simulink model "SimToStewartPlatform"  (R2020a)
settings: Solver=VariableStepAuto  StartTime=0.0  StopTime=inf  RelTol=1e-3
undefined symbols (not defined in the file or in its folder): Standard_Devices, UDP_Protocol
libraries: eeGeneralControl x3, instrumentlib x3, sldrtlib x1, simulink x1, ptplib x1
settings Model: xpc_rtwmakecfg_data=_xpcetherlib__xpcether8255xlib__xpcetherGbElib__xpciplib__xpcnblib_  Creator=meta_  LastModifiedBy=filip

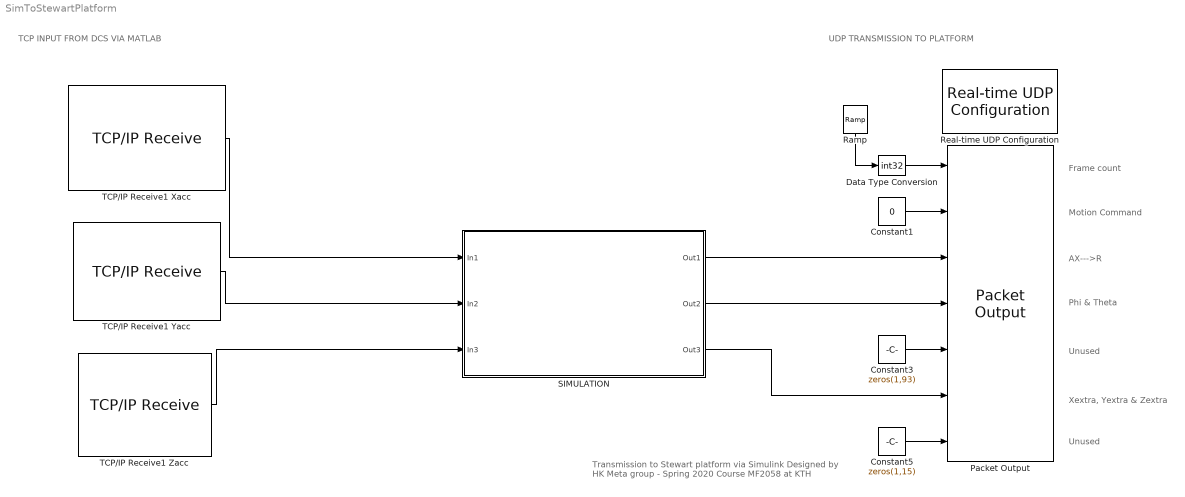
== system SimToStewartPlatform ==
  note: Transmission to Stewart platform via Simulink
      | Designed by HK Meta group - Spring 2020
      | Course MF2058 at KTH
  note: TCP INPUT FROM DCS VIA MATLAB
  note: UDP TRANSMISSION TO PLATFORM
  note: Unused
  note: Frame count
  note: Unused
  note: Phi & Theta
  note: Motion Command
  note: AX--->R
  note: Xextra, Yextra & Zextra
  Constant1 : Constant  Value=0
  Constant3 : Constant  Value=zeros(1,93)
  Constant5 : Constant  Value=zeros(1,15)
  Data Type Conversion : DataTypeConversion  OutDataTypeStr=int32
  Packet Output : sldrtlib/Packet Output  SampleTime=0.1  MaxMissedTicks=inf  ShowMissedTicks=off  YieldWhenWaiting=on  DrvName=Standard_Devices/UDP_Protocol  DrvAddress=16384  DrvOptions=[0 16385 49 57 50 46 49 54 56 46 57 48 46 50 52 48 0 0 0 0 0 0 0 0 0 0 0 0 0 0 0 0 0 0 0 0 0 0 0 0 0 0 0 0 0 0 0 0 0 0 0 0 0 0 0 0 0 0 0 0 0 0 0 0 0 0 0 0 0 0 0 0 0 0 0 0 0 0 0 0 0 0 0 0 0 0 0 0 0 0 0 0 0 0 0 0 0 0 0 0 0 0 0 0 0 0 0 0 0 0 0 0 0 0 0 0 0 0 0 0 0 0 0 0 0 0 0 0 0 0 0 0 0 0 0 0 0 0 0 0 0 0 0 0 0 0 0 0 0 0 0 0 0 0 0 0 0 0 0 0 0 0 0 0 0 0 0 0 0 0 0 0 0 0 0 0 0 0 0 0 0 0 0 0 0 0 0 0 0 0 0 0 0 0 0 0 0 0 0 0 0 0 0 0 0 0 0 0 0 0 0 0 0 0 0 0 0 0 0 0 0 0 0 0 0 0 0 0 0 0 0 0 0 0 0 0 0 0 0 0 0 0 0 0 0 0 0 0 0 0 0 0 0 0 0 0]  PacketSize=508  DataTypes={'1*int32','1*int32','12*single','2*single','93*single','3*single','15*single'}  ShowReady=off  ShowError=off  PacketID=1  ByteOrder=1  InitialValue=[]  FinalValue=[]
      settings: AttributesFormatString=UDP Protocol [16384]
  Ramp : simulink/Sources/Ramp  slope=10  start=0  InitialOutput=0
  "Real-time UDP Configuration " : ptplib/PTP UDP/Real-time UDP  Configuration   ID=1  IpAddress=192.168.90.241  SubnetMask=255.255.255.0  Gateway=0.0.0.0  EthDrv=Intel Gigabit  PciBus=0  PciSlot=31  PciFunction=6  udpID=0  MulticastList=[]  Multicast={}
      settings: SourceProductBaseCode=XP
  SIMULATION : Subsystem
  TCP/IP Receive1 Xacc : instrumentlib/TCP//IP Receive  Host=127.0.0.1  Port=31091  DataSize="[1  1]"  EnableBlockingMode=on  Timeout=10  SampleTime=0.01  DataType=ASCII  ByteOrder=BigEndian  ASCIIFormatting=%f  Terminator=LF
  TCP/IP Receive1 Yacc : instrumentlib/TCP//IP Receive  Host=127.0.0.1  Port=31092  DataSize="[1  1]"  EnableBlockingMode=on  Timeout=10  SampleTime=0.01  DataType=ASCII  ByteOrder=BigEndian  ASCIIFormatting=%f  Terminator=LF
  TCP/IP Receive1 Zacc : instrumentlib/TCP//IP Receive  Host=127.0.0.1  Port=31093  DataSize="[1  1]"  EnableBlockingMode=on  Timeout=10  SampleTime=0.01  DataType=ASCII  ByteOrder=BigEndian  ASCIIFormatting=%f  Terminator=LF
  wires:
  Data Type Conversion/1 -> Packet Output/1
  Constant5/1 -> Packet Output/7
  Constant3/1 -> Packet Output/5
  Ramp/1 -> Data Type Conversion/1
  Constant1/1 -> Packet Output/2
  TCP/IP Receive1 Xacc/1 -> SIMULATION/1(In1)
  TCP/IP Receive1 Yacc/1 -> SIMULATION/2(In2)
  TCP/IP Receive1 Zacc/1 -> SIMULATION/3(In3)
  SIMULATION/1(Out1) -> Packet Output/3
  SIMULATION/2(Out2) -> Packet Output/4
  SIMULATION/3(Out3) -> Packet Output/6

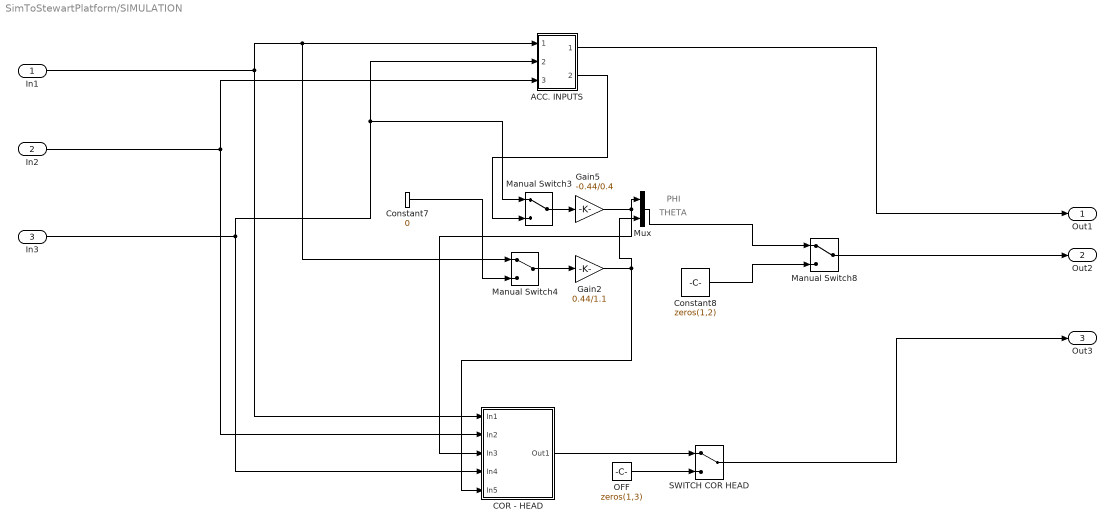
== system SimToStewartPlatform/SIMULATION ==
  note: THETA
  note: PHI
  In1 : Inport
  In2 : Inport  Port=2
  In3 : Inport  Port=3
  "ACC. INPUTS " : Subsystem
  COR - HEAD : Subsystem
  Constant7 : Constant  Value=0
  Constant8 : Constant  Value=zeros(1,2)
  Gain2 : Gain  Gain=0.44/1.1
  Gain5 : Gain  Gain=-0.44/0.4
  Manual Switch3 : ManualSwitch
  Manual Switch4 : ManualSwitch
  Manual Switch8 : ManualSwitch
  Mux : Mux  Inputs=2
  OFF : Constant  Value=zeros(1,3)
  SWITCH COR HEAD : ManualSwitch
  Out1 : Outport
  Out2 : Outport  Port=2
  Out3 : Outport  Port=3
  wires:
  COR - HEAD/1(Out1) -> SWITCH COR HEAD/1
  In1/1 -> COR - HEAD/1(In1), "ACC. INPUTS "/1(In1), Manual Switch4/1
  In3/1 -> COR - HEAD/4(In4), "ACC. INPUTS "/2(In2), Manual Switch3/1
  Gain5/1 -> COR - HEAD/3(In3), Mux/1
  Gain2/1 -> COR - HEAD/5(In5), Mux/2
  "ACC. INPUTS "/1(Out1) -> Out1/1
  Manual Switch3/1 -> Gain5/1
  Constant7/1 -> Manual Switch4/2
  Mux/1 -> Manual Switch8/1
  Constant8/1 -> Manual Switch8/2
  Manual Switch4/1 -> Gain2/1
  In2/1 -> "ACC. INPUTS "/3(In3), COR - HEAD/2(In2)
  SWITCH COR HEAD/1 -> Out3/1
  OFF/1 -> SWITCH COR HEAD/2
  "ACC. INPUTS "/2(Out2) -> Manual Switch3/2
  Manual Switch8/1 -> Out2/1

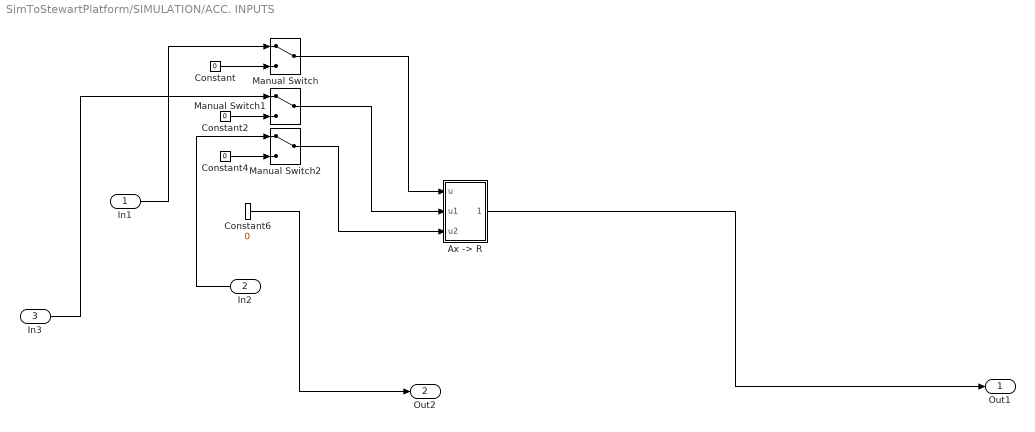
== system SimToStewartPlatform/SIMULATION/ACC. INPUTS  ==
  In1 : Inport
  In2 : Inport  Port=2
  In3 : Inport  Port=3
  "Ax -> R" : Subsystem
  Constant{,2,4,6} (4 alike) : Constant  Value=0
  Manual Switch : ManualSwitch
  Manual Switch1 : ManualSwitch
  Manual Switch2 : ManualSwitch
  Out1 : Outport
  Out2 : Outport  Port=2
  wires:
  Manual Switch2/1 -> "Ax -> R"/3(u2)
  "Ax -> R"/1(Out1) -> Out1/1
  Constant4/1 -> Manual Switch2/2
  Manual Switch/1 -> "Ax -> R"/1(u)
  Constant2/1 -> Manual Switch1/2
  In3/1 -> Manual Switch1/1
  Manual Switch1/1 -> "Ax -> R"/2(u1)
  Constant/1 -> Manual Switch/2
  In1/1 -> Manual Switch/1
  Constant6/1 -> Out2/1
  In2/1 -> Manual Switch2/1

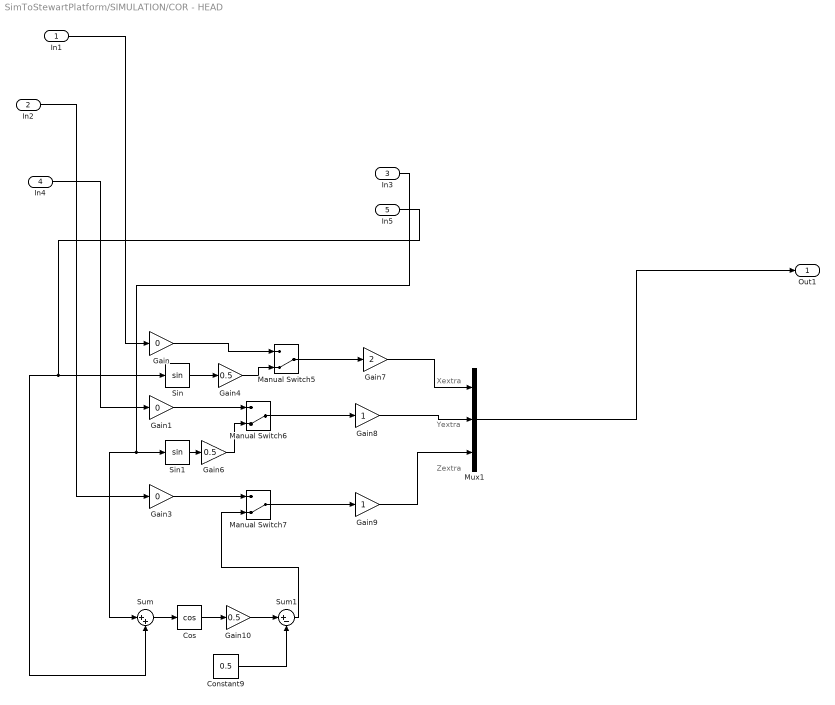
== system SimToStewartPlatform/SIMULATION/COR - HEAD ==
  note: Xextra
  note: Yextra
  note: Zextra
  In1 : Inport
  In2 : Inport  Port=2
  In3 : Inport  Port=3
  In4 : Inport  Port=4
  In5 : Inport  Port=5
  Constant9 : Constant  Value=0.5
  Cos : Trigonometry  Operator=cos
  Gain : Gain  Gain=0
  Gain1 : Gain  Gain=0
  Gain10 : Gain  Gain=0.5
  Gain3 : Gain  Gain=0
  Gain4 : Gain  Gain=0.5
  Gain6 : Gain  Gain=0.5
  Gain7 : Gain  Gain=2
  Gain8 : Gain
  Gain9 : Gain
  Manual Switch5 : ManualSwitch  CurrentSetting=0
  Manual Switch6 : ManualSwitch  CurrentSetting=0
  Manual Switch7 : ManualSwitch  CurrentSetting=0
  Mux1 : Mux  Inputs=3
  Sin : Trigonometry
  Sin1 : Trigonometry
  Sum : Sum  Inputs=|++
  Sum1 : Sum  Inputs=|+-
  Out1 : Outport
  wires:
  In3/1 -> Sum/1, Sin1/1
  Gain1/1 -> Manual Switch6/1
  In5/1 -> Sum/2, Sin/1
  Sin/1 -> Gain4/1
  Gain6/1 -> Manual Switch6/2
  Gain7/1 -> Mux1/1
  Sum/1 -> Cos/1
  Mux1/1 -> Out1/1
  Sin1/1 -> Gain6/1
  Gain/1 -> Manual Switch5/1
  Gain3/1 -> Manual Switch7/1
  Constant9/1 -> Sum1/2
  Sum1/1 -> Manual Switch7/2
  Gain9/1 -> Mux1/3
  Manual Switch5/1 -> Gain7/1
  Manual Switch7/1 -> Gain9/1
  Gain8/1 -> Mux1/2
  Cos/1 -> Gain10/1
  Gain4/1 -> Manual Switch5/2
  Manual Switch6/1 -> Gain8/1
  Gain10/1 -> Sum1/1
  In4/1 -> Gain1/1
  In2/1 -> Gain3/1
  In1/1 -> Gain/1

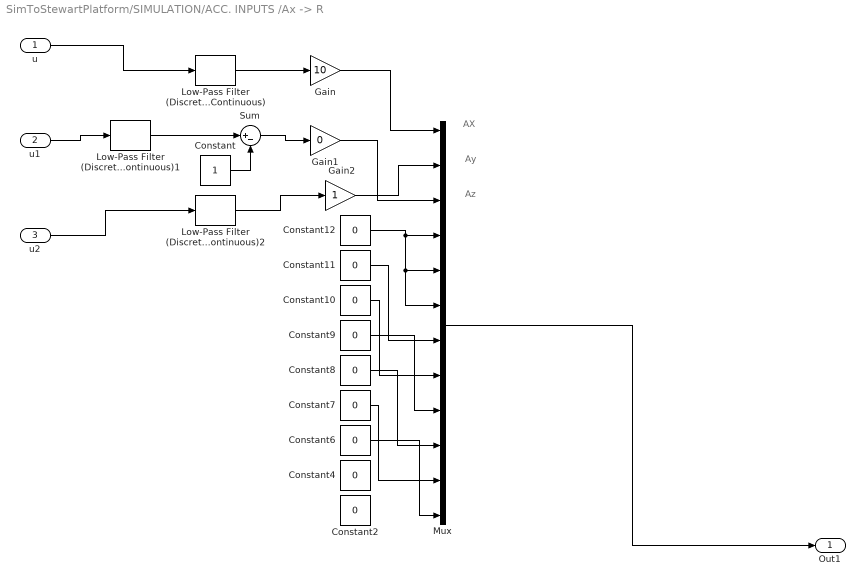
== system SimToStewartPlatform/SIMULATION/ACC. INPUTS /Ax -> R ==
  note: Az
  note: Ay
  note: AX
  u : Inport
  u1 : Inport  Port=2
  u2 : Inport  Port=3
  Constant : Constant
  Constant{2,4,6..12} (9 alike) : Constant  Value=0
  Gain : Gain  Gain=10
  Gain1 : Gain  Gain=0
  Gain2 : Gain
  Low-Pass Filter (Discrete or Continuous) : eeGeneralControl/Low-Pass Filter (Discrete or Continuous)  K=1  T=1  B=inf  A=-inf  init_option=Inherited from block input  x0=0  Ts=-1
  Low-Pass Filter (Discrete or Continuous)1 : eeGeneralControl/Low-Pass Filter (Discrete or Continuous)  K=1  T=1  B=inf  A=-inf  init_option=Inherited from block input  x0=0  Ts=-1
  Low-Pass Filter (Discrete or Continuous)2 : eeGeneralControl/Low-Pass Filter (Discrete or Continuous)  K=1  T=1  B=inf  A=-inf  init_option=Inherited from block input  x0=0  Ts=-1
  Mux : Mux  Inputs=12
  Sum : Sum  Inputs=|+-
  Out1 : Outport
  wires:
  Constant9/1 -> Mux/9
  u/1 -> Low-Pass Filter (Discrete or Continuous)/1
  Constant7/1 -> Mux/11
  u1/1 -> Low-Pass Filter (Discrete or Continuous)1/1
  Gain2/1 -> Mux/2
  Constant10/1 -> Mux/8
  Low-Pass Filter (Discrete or Continuous)2/1 -> Gain2/1
  Constant6/1 -> Mux/12
  Constant12/1 -> Mux/4, Mux/6, Mux/5
  Low-Pass Filter (Discrete or Continuous)/1 -> Gain/1
  Gain/1 -> Mux/1
  Constant11/1 -> Mux/7
  Constant8/1 -> Mux/10
  Gain1/1 -> Mux/3
  Low-Pass Filter (Discrete or Continuous)1/1 -> Sum/1
  Mux/1 -> Out1/1
  u2/1 -> Low-Pass Filter (Discrete or Continuous)2/1
  Constant/1 -> Sum/2
  Sum/1 -> Gain1/1
